simulink model "FOC_PMSM"  (Simulink 10.0)
settings: Solver=ode45  StartTime=0  StopTime=10  FixedStep=1/fs/4  MaxStep=1/fs/2  RelTol=1e-7  EnableMultiTasking=on
InitFcn:
  | Motor_parameters_Lsrpm7fw
values from neighbouring files (symbols this model uses):
  c2 = -L2/(L1^2-L2^2)    (= 10.9375)    [Motor_parameters_Lsrpm7fw.m]
  fs = 10e3    (= 10000)    [Motor_parameters_Lsrpm7fw.m]
  Iphmax = I_rated*sqrt(2)*3    [Motor_parameters_Lsrpm7fw.m]
  J = 1*1e-3    (= 0.001)    [Motor_parameters_Lsrpm7fw.m]
  Ki1 = 2    [Motor_parameters_Lsrpm7fw.m]
  Ki2 = 10000    [Motor_parameters_Lsrpm7fw.m]
  Ki_pll = 100    [Motor_parameters_Lsrpm7fw.m]
  Kp1 = 0.05    [Motor_parameters_Lsrpm7fw.m]
  Kp2 = 12    [Motor_parameters_Lsrpm7fw.m]
  Kp_pll = 10    [Motor_parameters_Lsrpm7fw.m]
  Ld = 10e-3    (= 0.01)    [Motor_parameters_Lsrpm7fw.m]
  Lndd_ini = Lndmpm    (= 0.412)    [Motor_parameters_Lsrpm7fw.m]
  Lndmpm = 0.412    [Motor_parameters_Lsrpm7fw.m]
  Lq = 12.8e-3    (= 0.0128)    [Motor_parameters_Lsrpm7fw.m]
  Npp = 8/2    (= 4)    [Motor_parameters_Lsrpm7fw.m]
  Omegae_ini = 0    [Motor_parameters_Lsrpm7fw.m]
  Rs = 0.78    [Motor_parameters_Lsrpm7fw.m]
  Tl_const = Trat/nrat^2    (= 1.24081632653e-05)    [Motor_parameters_Lsrpm7fw.m]
  Trat = 38    [Motor_parameters_Lsrpm7fw.m]
  Vm = 45    [Motor_parameters_Lsrpm7fw.m]
  Vph = Vs*sqrt(2)    [Motor_parameters_Lsrpm7fw.m]
  wo = 10    [Motor_parameters_Lsrpm7fw.m]
undefined symbols (not defined in the file or in its folder): DiscIntNeverNeededParam, sigbuilder_block
libraries: simulink x1
(part 2 of 2)

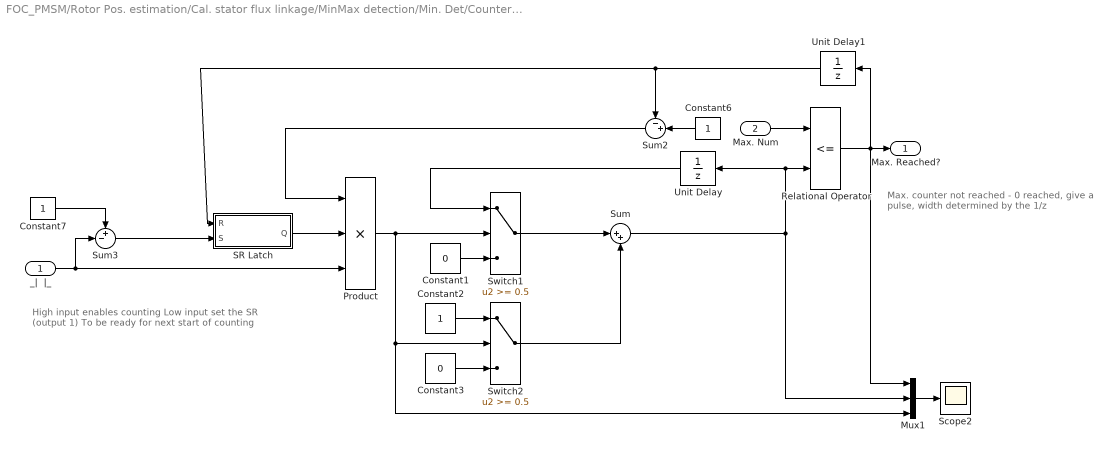
== system FOC_PMSM/Rotor Pos. estimation/Cal. stator flux linkage/MinMax detection/Min. Det/Counter.1/Conter with enable ==
  note: Max. counter not reached - 0
      | reached, give a pulse, width
      | determined by the 1/z
  note: High input enables counting
      | Low input set the SR (output 1)
      | To be ready for next start of
      | counting
  _|  |_ : Inport
  Max. Num : Inport  Port=2
  Constant1 : Constant  Value=0
  Constant2 : Constant
  Constant3 : Constant  Value=0
  Constant6 : Constant
  Constant7 : Constant
  Mux1 : Mux  Inputs=3
  Product : Product  Inputs=3  RndMeth=Zero
  Relational Operator : RelationalOperator  Operator=<=  RndMeth=Nearest
  SR Latch : Subsystem
  Scope2 : Scope
  Sum : Sum  Inputs=|++
  Sum2 : Sum  Inputs=-+|
  Sum3 : Sum  Inputs=+-|
  Switch1 : Switch  Threshold=0.5
  Switch2 : Switch  Threshold=0.5
  Unit Delay : UnitDelay  SampleTime=-1  HasFrameUpgradeWarning=on
  Unit Delay1 : UnitDelay  SampleTime=-1  HasFrameUpgradeWarning=on
  Max. Reached? : Outport  VectorParamsAs1DForOutWhenUnconnected=off
  wires:
  Unit Delay1/1 -> SR Latch/1(R), Sum2/1
  Constant6/1 -> Sum2/2
  Constant7/1 -> Sum3/1
  Sum3/1 -> SR Latch/2(S)
  SR Latch/1(Q) -> Product/2
  _|  |_/1 -> Product/3, Sum3/2
  Product/1 -> Mux1/3, Switch2/2, Switch1/2
  Sum2/1 -> Product/1
  Mux1/1 -> Scope2/1
  Relational Operator/1 -> Max. Reached?/1, Unit Delay1/1, Mux1/1
  Max. Num/1 -> Relational Operator/1
  Unit Delay/1 -> Switch1/1
  Sum/1 -> Mux1/2, Relational Operator/2, Unit Delay/1
  Switch2/1 -> Sum/2
  Switch1/1 -> Sum/1
  Constant3/1 -> Switch2/3
  Constant2/1 -> Switch2/1
  Constant1/1 -> Switch1/3

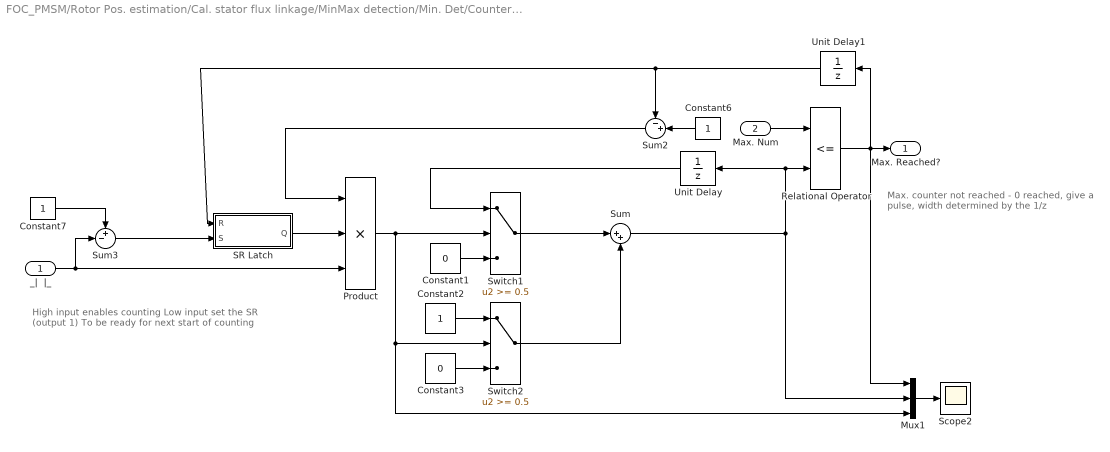
== system FOC_PMSM/Rotor Pos. estimation/Cal. stator flux linkage/MinMax detection/Min. Det/Counter.2/Conter with enable ==
  note: High input enables counting
      | Low input set the SR (output 1)
      | To be ready for next start of
      | counting
  note: Max. counter not reached - 0
      | reached, give a pulse, width
      | determined by the 1/z
  _|  |_ : Inport
  Max. Num : Inport  Port=2
  Constant1 : Constant  Value=0
  Constant2 : Constant
  Constant3 : Constant  Value=0
  Constant6 : Constant
  Constant7 : Constant
  Mux1 : Mux  Inputs=3
  Product : Product  Inputs=3  RndMeth=Zero
  Relational Operator : RelationalOperator  Operator=<=  RndMeth=Nearest
  SR Latch : Subsystem
  Scope2 : Scope
  Sum : Sum  Inputs=|++
  Sum2 : Sum  Inputs=-+|
  Sum3 : Sum  Inputs=+-|
  Switch1 : Switch  Threshold=0.5
  Switch2 : Switch  Threshold=0.5
  Unit Delay : UnitDelay  SampleTime=-1  HasFrameUpgradeWarning=on
  Unit Delay1 : UnitDelay  SampleTime=-1  HasFrameUpgradeWarning=on
  Max. Reached? : Outport  VectorParamsAs1DForOutWhenUnconnected=off
  wires:
  Constant1/1 -> Switch1/3
  Constant2/1 -> Switch2/1
  Constant3/1 -> Switch2/3
  Switch1/1 -> Sum/1
  Switch2/1 -> Sum/2
  Sum/1 -> Unit Delay/1, Relational Operator/2, Mux1/2
  Unit Delay/1 -> Switch1/1
  Max. Num/1 -> Relational Operator/1
  Relational Operator/1 -> Mux1/1, Unit Delay1/1, Max. Reached?/1
  Mux1/1 -> Scope2/1
  Sum2/1 -> Product/1
  Product/1 -> Switch1/2, Switch2/2, Mux1/3
  _|  |_/1 -> Sum3/2, Product/3
  SR Latch/1(Q) -> Product/2
  Sum3/1 -> SR Latch/2(S)
  Constant7/1 -> Sum3/1
  Constant6/1 -> Sum2/2
  Unit Delay1/1 -> Sum2/1, SR Latch/1(R)

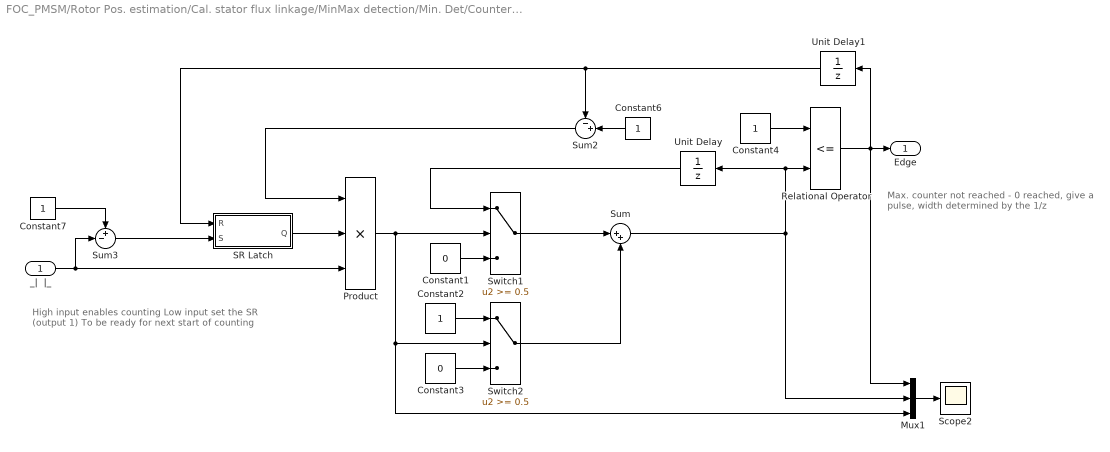
== system FOC_PMSM/Rotor Pos. estimation/Cal. stator flux linkage/MinMax detection/Min. Det/Counter.2/Rising edge gen. ==
  note: Max. counter not reached - 0
      | reached, give a pulse, width
      | determined by the 1/z
  note: High input enables counting
      | Low input set the SR (output 1)
      | To be ready for next start of
      | counting
  _|  |_ : Inport
  Constant1 : Constant  Value=0
  Constant{2,4,6..7} (4 alike) : Constant
  Constant3 : Constant  Value=0
  Mux1 : Mux  Inputs=3
  Product : Product  Inputs=3  RndMeth=Zero
  Relational Operator : RelationalOperator  Operator=<=  RndMeth=Nearest
  SR Latch : Subsystem
  Scope2 : Scope
  Sum : Sum  Inputs=|++
  Sum2 : Sum  Inputs=-+|
  Sum3 : Sum  Inputs=+-|
  Switch1 : Switch  Threshold=0.5
  Switch2 : Switch  Threshold=0.5
  Unit Delay : UnitDelay  SampleTime=-1  HasFrameUpgradeWarning=on
  Unit Delay1 : UnitDelay  SampleTime=-1  HasFrameUpgradeWarning=on
  Edge : Outport  VectorParamsAs1DForOutWhenUnconnected=off
  wires:
  Unit Delay1/1 -> SR Latch/1(R), Sum2/1
  Constant6/1 -> Sum2/2
  Constant7/1 -> Sum3/1
  Sum3/1 -> SR Latch/2(S)
  SR Latch/1(Q) -> Product/2
  _|  |_/1 -> Product/3, Sum3/2
  Product/1 -> Mux1/3, Switch2/2, Switch1/2
  Sum2/1 -> Product/1
  Mux1/1 -> Scope2/1
  Relational Operator/1 -> Edge/1, Unit Delay1/1, Mux1/1
  Constant4/1 -> Relational Operator/1
  Unit Delay/1 -> Switch1/1
  Sum/1 -> Mux1/2, Relational Operator/2, Unit Delay/1
  Switch2/1 -> Sum/2
  Switch1/1 -> Sum/1
  Constant3/1 -> Switch2/3
  Constant2/1 -> Switch2/1
  Constant1/1 -> Switch1/3

== system FOC_PMSM/Rotor Pos. estimation/Cal. stator flux linkage/MinMax detection/Min. Det/Counter.2/SR Latch ==
  R : Inport
  S : Inport  Port=2
  Constant2 : Constant
  Constant4 : Constant  Value=0
  Constant5 : Constant  Value=0
  Multiport Switch : MultiPortSwitch  Inputs=4
  Mux1 : Mux  Inputs=2
  Selcect : Fcn  Expr=(1-u(1))*(1-u(2))+2*(1-u(1))*u(2)+3*u(1)*(1-u(2))+4*u(1)*u(2)
  Unit Delay2 : UnitDelay  SampleTime=-1  HasFrameUpgradeWarning=on
  Q : Outport  VectorParamsAs1DForOutWhenUnconnected=off
  wires:
  Multiport Switch/1 -> Q/1, Unit Delay2/1
  Selcect/1 -> Multiport Switch/1
  Mux1/1 -> Selcect/1
  Unit Delay2/1 -> Multiport Switch/2
  Constant2/1 -> Multiport Switch/3
  Constant4/1 -> Multiport Switch/4
  Constant5/1 -> Multiport Switch/5
  R/1 -> Mux1/1
  S/1 -> Mux1/2

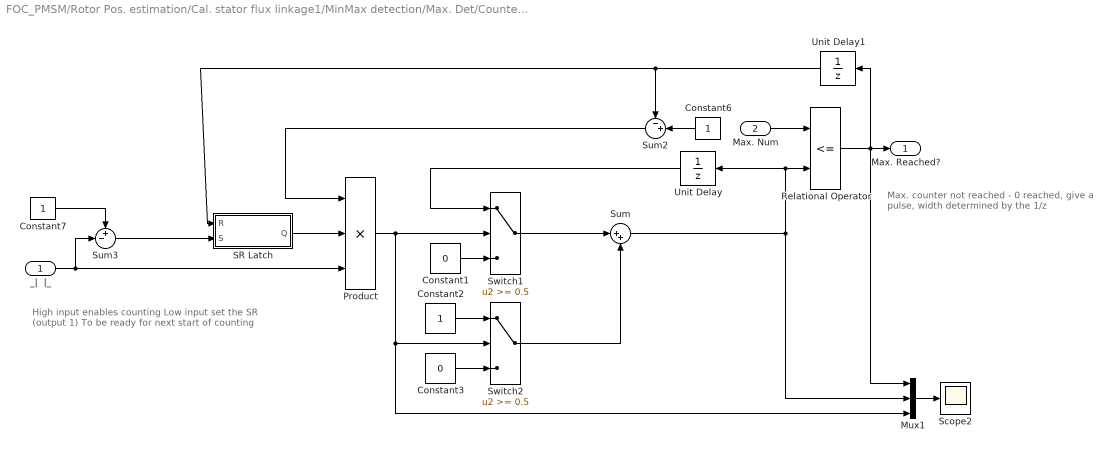
== system FOC_PMSM/Rotor Pos. estimation/Cal. stator flux linkage1/MinMax detection/Max. Det/Counter.1/Conter with enable ==
  note: High input enables counting
      | Low input set the SR (output 1)
      | To be ready for next start of
      | counting
  note: Max. counter not reached - 0
      | reached, give a pulse, width
      | determined by the 1/z
  _|  |_ : Inport
  Max. Num : Inport  Port=2
  Constant1 : Constant  Value=0
  Constant2 : Constant
  Constant3 : Constant  Value=0
  Constant6 : Constant
  Constant7 : Constant
  Mux1 : Mux  Inputs=3
  Product : Product  Inputs=3  RndMeth=Zero
  Relational Operator : RelationalOperator  Operator=<=  RndMeth=Nearest
  SR Latch : Subsystem
  Scope2 : Scope
  Sum : Sum  Inputs=|++
  Sum2 : Sum  Inputs=-+|
  Sum3 : Sum  Inputs=+-|
  Switch1 : Switch  Threshold=0.5
  Switch2 : Switch  Threshold=0.5
  Unit Delay : UnitDelay  SampleTime=-1  HasFrameUpgradeWarning=on
  Unit Delay1 : UnitDelay  SampleTime=-1  HasFrameUpgradeWarning=on
  Max. Reached? : Outport  VectorParamsAs1DForOutWhenUnconnected=off
  wires:
  Constant1/1 -> Switch1/3
  Constant2/1 -> Switch2/1
  Constant3/1 -> Switch2/3
  Switch1/1 -> Sum/1
  Switch2/1 -> Sum/2
  Sum/1 -> Unit Delay/1, Relational Operator/2, Mux1/2
  Unit Delay/1 -> Switch1/1
  Max. Num/1 -> Relational Operator/1
  Relational Operator/1 -> Mux1/1, Unit Delay1/1, Max. Reached?/1
  Mux1/1 -> Scope2/1
  Sum2/1 -> Product/1
  Product/1 -> Switch1/2, Switch2/2, Mux1/3
  _|  |_/1 -> Sum3/2, Product/3
  SR Latch/1(Q) -> Product/2
  Sum3/1 -> SR Latch/2(S)
  Constant7/1 -> Sum3/1
  Constant6/1 -> Sum2/2
  Unit Delay1/1 -> Sum2/1, SR Latch/1(R)

== system FOC_PMSM/Rotor Pos. estimation/Cal. stator flux linkage1/MinMax detection/Max. Det/Counter.2/Conter with enable ==
  note: Max. counter not reached - 0
      | reached, give a pulse, width
      | determined by the 1/z
  note: High input enables counting
      | Low input set the SR (output 1)
      | To be ready for next start of
      | counting
  _|  |_ : Inport
  Max. Num : Inport  Port=2
  Constant1 : Constant  Value=0
  Constant2 : Constant
  Constant3 : Constant  Value=0
  Constant6 : Constant
  Constant7 : Constant
  Mux1 : Mux  Inputs=3
  Product : Product  Inputs=3  RndMeth=Zero
  Relational Operator : RelationalOperator  Operator=<=  RndMeth=Nearest
  SR Latch : Subsystem
  Scope2 : Scope
  Sum : Sum  Inputs=|++
  Sum2 : Sum  Inputs=-+|
  Sum3 : Sum  Inputs=+-|
  Switch1 : Switch  Threshold=0.5
  Switch2 : Switch  Threshold=0.5
  Unit Delay : UnitDelay  SampleTime=-1  HasFrameUpgradeWarning=on
  Unit Delay1 : UnitDelay  SampleTime=-1  HasFrameUpgradeWarning=on
  Max. Reached? : Outport  VectorParamsAs1DForOutWhenUnconnected=off
  wires:
  Unit Delay1/1 -> SR Latch/1(R), Sum2/1
  Constant6/1 -> Sum2/2
  Constant7/1 -> Sum3/1
  Sum3/1 -> SR Latch/2(S)
  SR Latch/1(Q) -> Product/2
  _|  |_/1 -> Product/3, Sum3/2
  Product/1 -> Mux1/3, Switch2/2, Switch1/2
  Sum2/1 -> Product/1
  Mux1/1 -> Scope2/1
  Relational Operator/1 -> Max. Reached?/1, Unit Delay1/1, Mux1/1
  Max. Num/1 -> Relational Operator/1
  Unit Delay/1 -> Switch1/1
  Sum/1 -> Mux1/2, Relational Operator/2, Unit Delay/1
  Switch2/1 -> Sum/2
  Switch1/1 -> Sum/1
  Constant3/1 -> Switch2/3
  Constant2/1 -> Switch2/1
  Constant1/1 -> Switch1/3

== system FOC_PMSM/Rotor Pos. estimation/Cal. stator flux linkage1/MinMax detection/Max. Det/Counter.2/Rising edge gen. ==
  note: High input enables counting
      | Low input set the SR (output 1)
      | To be ready for next start of
      | counting
  note: Max. counter not reached - 0
      | reached, give a pulse, width
      | determined by the 1/z
  _|  |_ : Inport
  Constant1 : Constant  Value=0
  Constant{2,4,6..7} (4 alike) : Constant
  Constant3 : Constant  Value=0
  Mux1 : Mux  Inputs=3
  Product : Product  Inputs=3  RndMeth=Zero
  Relational Operator : RelationalOperator  Operator=<=  RndMeth=Nearest
  SR Latch : Subsystem
  Scope2 : Scope
  Sum : Sum  Inputs=|++
  Sum2 : Sum  Inputs=-+|
  Sum3 : Sum  Inputs=+-|
  Switch1 : Switch  Threshold=0.5
  Switch2 : Switch  Threshold=0.5
  Unit Delay : UnitDelay  SampleTime=-1  HasFrameUpgradeWarning=on
  Unit Delay1 : UnitDelay  SampleTime=-1  HasFrameUpgradeWarning=on
  Edge : Outport  VectorParamsAs1DForOutWhenUnconnected=off
  wires:
  Constant1/1 -> Switch1/3
  Constant2/1 -> Switch2/1
  Constant3/1 -> Switch2/3
  Switch1/1 -> Sum/1
  Switch2/1 -> Sum/2
  Sum/1 -> Unit Delay/1, Relational Operator/2, Mux1/2
  Unit Delay/1 -> Switch1/1
  Constant4/1 -> Relational Operator/1
  Relational Operator/1 -> Mux1/1, Unit Delay1/1, Edge/1
  Mux1/1 -> Scope2/1
  Sum2/1 -> Product/1
  Product/1 -> Switch1/2, Switch2/2, Mux1/3
  _|  |_/1 -> Sum3/2, Product/3
  SR Latch/1(Q) -> Product/2
  Sum3/1 -> SR Latch/2(S)
  Constant7/1 -> Sum3/1
  Constant6/1 -> Sum2/2
  Unit Delay1/1 -> Sum2/1, SR Latch/1(R)

== system FOC_PMSM/Rotor Pos. estimation/Cal. stator flux linkage1/MinMax detection/Max. Det/Counter.2/SR Latch ==
  R : Inport
  S : Inport  Port=2
  Constant2 : Constant
  Constant4 : Constant  Value=0
  Constant5 : Constant  Value=0
  Multiport Switch : MultiPortSwitch  Inputs=4
  Mux1 : Mux  Inputs=2
  Selcect : Fcn  Expr=(1-u(1))*(1-u(2))+2*(1-u(1))*u(2)+3*u(1)*(1-u(2))+4*u(1)*u(2)
  Unit Delay2 : UnitDelay  SampleTime=-1  HasFrameUpgradeWarning=on
  Q : Outport  VectorParamsAs1DForOutWhenUnconnected=off
  wires:
  S/1 -> Mux1/2
  R/1 -> Mux1/1
  Constant5/1 -> Multiport Switch/5
  Constant4/1 -> Multiport Switch/4
  Constant2/1 -> Multiport Switch/3
  Unit Delay2/1 -> Multiport Switch/2
  Mux1/1 -> Selcect/1
  Selcect/1 -> Multiport Switch/1
  Multiport Switch/1 -> Unit Delay2/1, Q/1

== system FOC_PMSM/Rotor Pos. estimation/Cal. stator flux linkage1/MinMax detection/Min. Det/Counter.1/Conter with enable ==
  note: Max. counter not reached - 0
      | reached, give a pulse, width
      | determined by the 1/z
  note: High input enables counting
      | Low input set the SR (output 1)
      | To be ready for next start of
      | counting
  _|  |_ : Inport
  Max. Num : Inport  Port=2
  Constant1 : Constant  Value=0
  Constant2 : Constant
  Constant3 : Constant  Value=0
  Constant6 : Constant
  Constant7 : Constant
  Mux1 : Mux  Inputs=3
  Product : Product  Inputs=3  RndMeth=Zero
  Relational Operator : RelationalOperator  Operator=<=  RndMeth=Nearest
  SR Latch : Subsystem
  Scope2 : Scope
  Sum : Sum  Inputs=|++
  Sum2 : Sum  Inputs=-+|
  Sum3 : Sum  Inputs=+-|
  Switch1 : Switch  Threshold=0.5
  Switch2 : Switch  Threshold=0.5
  Unit Delay : UnitDelay  SampleTime=-1  HasFrameUpgradeWarning=on
  Unit Delay1 : UnitDelay  SampleTime=-1  HasFrameUpgradeWarning=on
  Max. Reached? : Outport  VectorParamsAs1DForOutWhenUnconnected=off
  wires:
  Unit Delay1/1 -> SR Latch/1(R), Sum2/1
  Constant6/1 -> Sum2/2
  Constant7/1 -> Sum3/1
  Sum3/1 -> SR Latch/2(S)
  SR Latch/1(Q) -> Product/2
  _|  |_/1 -> Product/3, Sum3/2
  Product/1 -> Mux1/3, Switch2/2, Switch1/2
  Sum2/1 -> Product/1
  Mux1/1 -> Scope2/1
  Relational Operator/1 -> Max. Reached?/1, Unit Delay1/1, Mux1/1
  Max. Num/1 -> Relational Operator/1
  Unit Delay/1 -> Switch1/1
  Sum/1 -> Mux1/2, Relational Operator/2, Unit Delay/1
  Switch2/1 -> Sum/2
  Switch1/1 -> Sum/1
  Constant3/1 -> Switch2/3
  Constant2/1 -> Switch2/1
  Constant1/1 -> Switch1/3

== system FOC_PMSM/Rotor Pos. estimation/Cal. stator flux linkage1/MinMax detection/Min. Det/Counter.2/Conter with enable ==
  note: High input enables counting
      | Low input set the SR (output 1)
      | To be ready for next start of
      | counting
  note: Max. counter not reached - 0
      | reached, give a pulse, width
      | determined by the 1/z
  _|  |_ : Inport
  Max. Num : Inport  Port=2
  Constant1 : Constant  Value=0
  Constant2 : Constant
  Constant3 : Constant  Value=0
  Constant6 : Constant
  Constant7 : Constant
  Mux1 : Mux  Inputs=3
  Product : Product  Inputs=3  RndMeth=Zero
  Relational Operator : RelationalOperator  Operator=<=  RndMeth=Nearest
  SR Latch : Subsystem
  Scope2 : Scope
  Sum : Sum  Inputs=|++
  Sum2 : Sum  Inputs=-+|
  Sum3 : Sum  Inputs=+-|
  Switch1 : Switch  Threshold=0.5
  Switch2 : Switch  Threshold=0.5
  Unit Delay : UnitDelay  SampleTime=-1  HasFrameUpgradeWarning=on
  Unit Delay1 : UnitDelay  SampleTime=-1  HasFrameUpgradeWarning=on
  Max. Reached? : Outport  VectorParamsAs1DForOutWhenUnconnected=off
  wires:
  Constant1/1 -> Switch1/3
  Constant2/1 -> Switch2/1
  Constant3/1 -> Switch2/3
  Switch1/1 -> Sum/1
  Switch2/1 -> Sum/2
  Sum/1 -> Unit Delay/1, Relational Operator/2, Mux1/2
  Unit Delay/1 -> Switch1/1
  Max. Num/1 -> Relational Operator/1
  Relational Operator/1 -> Mux1/1, Unit Delay1/1, Max. Reached?/1
  Mux1/1 -> Scope2/1
  Sum2/1 -> Product/1
  Product/1 -> Switch1/2, Switch2/2, Mux1/3
  _|  |_/1 -> Sum3/2, Product/3
  SR Latch/1(Q) -> Product/2
  Sum3/1 -> SR Latch/2(S)
  Constant7/1 -> Sum3/1
  Constant6/1 -> Sum2/2
  Unit Delay1/1 -> Sum2/1, SR Latch/1(R)

== system FOC_PMSM/Rotor Pos. estimation/Cal. stator flux linkage1/MinMax detection/Min. Det/Counter.2/Rising edge gen. ==
  note: Max. counter not reached - 0
      | reached, give a pulse, width
      | determined by the 1/z
  note: High input enables counting
      | Low input set the SR (output 1)
      | To be ready for next start of
      | counting
  _|  |_ : Inport
  Constant1 : Constant  Value=0
  Constant{2,4,6..7} (4 alike) : Constant
  Constant3 : Constant  Value=0
  Mux1 : Mux  Inputs=3
  Product : Product  Inputs=3  RndMeth=Zero
  Relational Operator : RelationalOperator  Operator=<=  RndMeth=Nearest
  SR Latch : Subsystem
  Scope2 : Scope
  Sum : Sum  Inputs=|++
  Sum2 : Sum  Inputs=-+|
  Sum3 : Sum  Inputs=+-|
  Switch1 : Switch  Threshold=0.5
  Switch2 : Switch  Threshold=0.5
  Unit Delay : UnitDelay  SampleTime=-1  HasFrameUpgradeWarning=on
  Unit Delay1 : UnitDelay  SampleTime=-1  HasFrameUpgradeWarning=on
  Edge : Outport  VectorParamsAs1DForOutWhenUnconnected=off
  wires:
  Unit Delay1/1 -> SR Latch/1(R), Sum2/1
  Constant6/1 -> Sum2/2
  Constant7/1 -> Sum3/1
  Sum3/1 -> SR Latch/2(S)
  SR Latch/1(Q) -> Product/2
  _|  |_/1 -> Product/3, Sum3/2
  Product/1 -> Mux1/3, Switch2/2, Switch1/2
  Sum2/1 -> Product/1
  Mux1/1 -> Scope2/1
  Relational Operator/1 -> Edge/1, Unit Delay1/1, Mux1/1
  Constant4/1 -> Relational Operator/1
  Unit Delay/1 -> Switch1/1
  Sum/1 -> Mux1/2, Relational Operator/2, Unit Delay/1
  Switch2/1 -> Sum/2
  Switch1/1 -> Sum/1
  Constant3/1 -> Switch2/3
  Constant2/1 -> Switch2/1
  Constant1/1 -> Switch1/3

== system FOC_PMSM/Rotor Pos. estimation/Cal. stator flux linkage1/MinMax detection/Min. Det/Counter.2/SR Latch ==
  R : Inport
  S : Inport  Port=2
  Constant2 : Constant
  Constant4 : Constant  Value=0
  Constant5 : Constant  Value=0
  Multiport Switch : MultiPortSwitch  Inputs=4
  Mux1 : Mux  Inputs=2
  Selcect : Fcn  Expr=(1-u(1))*(1-u(2))+2*(1-u(1))*u(2)+3*u(1)*(1-u(2))+4*u(1)*u(2)
  Unit Delay2 : UnitDelay  SampleTime=-1  HasFrameUpgradeWarning=on
  Q : Outport  VectorParamsAs1DForOutWhenUnconnected=off
  wires:
  Multiport Switch/1 -> Q/1, Unit Delay2/1
  Selcect/1 -> Multiport Switch/1
  Mux1/1 -> Selcect/1
  Unit Delay2/1 -> Multiport Switch/2
  Constant2/1 -> Multiport Switch/3
  Constant4/1 -> Multiport Switch/4
  Constant5/1 -> Multiport Switch/5
  R/1 -> Mux1/1
  S/1 -> Mux1/2

== system FOC_PMSM/Rotor Pos. estimation/Cal. stator flux linkage/MinMax detection/Max. Det/Counter.1/Conter with enable/SR Latch ==
  R : Inport
  S : Inport  Port=2
  Constant2 : Constant
  Constant4 : Constant  Value=0
  Constant5 : Constant  Value=0
  Multiport Switch : MultiPortSwitch  Inputs=4
  Mux1 : Mux  Inputs=2
  Selcect : Fcn  Expr=(1-u(1))*(1-u(2))+2*(1-u(1))*u(2)+3*u(1)*(1-u(2))+4*u(1)*u(2)
  Unit Delay2 : UnitDelay  SampleTime=-1  HasFrameUpgradeWarning=on
  Q : Outport  VectorParamsAs1DForOutWhenUnconnected=off
  wires:
  Multiport Switch/1 -> Q/1, Unit Delay2/1
  Selcect/1 -> Multiport Switch/1
  Mux1/1 -> Selcect/1
  Unit Delay2/1 -> Multiport Switch/2
  Constant2/1 -> Multiport Switch/3
  Constant4/1 -> Multiport Switch/4
  Constant5/1 -> Multiport Switch/5
  R/1 -> Mux1/1
  S/1 -> Mux1/2

== system FOC_PMSM/Rotor Pos. estimation/Cal. stator flux linkage/MinMax detection/Max. Det/Counter.2/Conter with enable/SR Latch ==
  R : Inport
  S : Inport  Port=2
  Constant2 : Constant
  Constant4 : Constant  Value=0
  Constant5 : Constant  Value=0
  Multiport Switch : MultiPortSwitch  Inputs=4
  Mux1 : Mux  Inputs=2
  Selcect : Fcn  Expr=(1-u(1))*(1-u(2))+2*(1-u(1))*u(2)+3*u(1)*(1-u(2))+4*u(1)*u(2)
  Unit Delay2 : UnitDelay  SampleTime=-1  HasFrameUpgradeWarning=on
  Q : Outport  VectorParamsAs1DForOutWhenUnconnected=off
  wires:
  S/1 -> Mux1/2
  R/1 -> Mux1/1
  Constant5/1 -> Multiport Switch/5
  Constant4/1 -> Multiport Switch/4
  Constant2/1 -> Multiport Switch/3
  Unit Delay2/1 -> Multiport Switch/2
  Mux1/1 -> Selcect/1
  Selcect/1 -> Multiport Switch/1
  Multiport Switch/1 -> Unit Delay2/1, Q/1

== system FOC_PMSM/Rotor Pos. estimation/Cal. stator flux linkage/MinMax detection/Max. Det/Counter.2/Rising edge gen./SR Latch ==
  R : Inport
  S : Inport  Port=2
  Constant2 : Constant
  Constant4 : Constant  Value=0
  Constant5 : Constant  Value=0
  Multiport Switch : MultiPortSwitch  Inputs=4
  Mux1 : Mux  Inputs=2
  Selcect : Fcn  Expr=(1-u(1))*(1-u(2))+2*(1-u(1))*u(2)+3*u(1)*(1-u(2))+4*u(1)*u(2)
  Unit Delay2 : UnitDelay  SampleTime=-1  HasFrameUpgradeWarning=on
  Q : Outport  VectorParamsAs1DForOutWhenUnconnected=off
  wires:
  Multiport Switch/1 -> Q/1, Unit Delay2/1
  Selcect/1 -> Multiport Switch/1
  Mux1/1 -> Selcect/1
  Unit Delay2/1 -> Multiport Switch/2
  Constant2/1 -> Multiport Switch/3
  Constant4/1 -> Multiport Switch/4
  Constant5/1 -> Multiport Switch/5
  R/1 -> Mux1/1
  S/1 -> Mux1/2

== system FOC_PMSM/Rotor Pos. estimation/Cal. stator flux linkage/MinMax detection/Min. Det/Counter.1/Conter with enable/SR Latch ==
  R : Inport
  S : Inport  Port=2
  Constant2 : Constant
  Constant4 : Constant  Value=0
  Constant5 : Constant  Value=0
  Multiport Switch : MultiPortSwitch  Inputs=4
  Mux1 : Mux  Inputs=2
  Selcect : Fcn  Expr=(1-u(1))*(1-u(2))+2*(1-u(1))*u(2)+3*u(1)*(1-u(2))+4*u(1)*u(2)
  Unit Delay2 : UnitDelay  SampleTime=-1  HasFrameUpgradeWarning=on
  Q : Outport  VectorParamsAs1DForOutWhenUnconnected=off
  wires:
  S/1 -> Mux1/2
  R/1 -> Mux1/1
  Constant5/1 -> Multiport Switch/5
  Constant4/1 -> Multiport Switch/4
  Constant2/1 -> Multiport Switch/3
  Unit Delay2/1 -> Multiport Switch/2
  Mux1/1 -> Selcect/1
  Selcect/1 -> Multiport Switch/1
  Multiport Switch/1 -> Unit Delay2/1, Q/1

== system FOC_PMSM/Rotor Pos. estimation/Cal. stator flux linkage/MinMax detection/Min. Det/Counter.2/Conter with enable/SR Latch ==
  R : Inport
  S : Inport  Port=2
  Constant2 : Constant
  Constant4 : Constant  Value=0
  Constant5 : Constant  Value=0
  Multiport Switch : MultiPortSwitch  Inputs=4
  Mux1 : Mux  Inputs=2
  Selcect : Fcn  Expr=(1-u(1))*(1-u(2))+2*(1-u(1))*u(2)+3*u(1)*(1-u(2))+4*u(1)*u(2)
  Unit Delay2 : UnitDelay  SampleTime=-1  HasFrameUpgradeWarning=on
  Q : Outport  VectorParamsAs1DForOutWhenUnconnected=off
  wires:
  Multiport Switch/1 -> Q/1, Unit Delay2/1
  Selcect/1 -> Multiport Switch/1
  Mux1/1 -> Selcect/1
  Unit Delay2/1 -> Multiport Switch/2
  Constant2/1 -> Multiport Switch/3
  Constant4/1 -> Multiport Switch/4
  Constant5/1 -> Multiport Switch/5
  R/1 -> Mux1/1
  S/1 -> Mux1/2

== system FOC_PMSM/Rotor Pos. estimation/Cal. stator flux linkage/MinMax detection/Min. Det/Counter.2/Rising edge gen./SR Latch ==
  R : Inport
  S : Inport  Port=2
  Constant2 : Constant
  Constant4 : Constant  Value=0
  Constant5 : Constant  Value=0
  Multiport Switch : MultiPortSwitch  Inputs=4
  Mux1 : Mux  Inputs=2
  Selcect : Fcn  Expr=(1-u(1))*(1-u(2))+2*(1-u(1))*u(2)+3*u(1)*(1-u(2))+4*u(1)*u(2)
  Unit Delay2 : UnitDelay  SampleTime=-1  HasFrameUpgradeWarning=on
  Q : Outport  VectorParamsAs1DForOutWhenUnconnected=off
  wires:
  S/1 -> Mux1/2
  R/1 -> Mux1/1
  Constant5/1 -> Multiport Switch/5
  Constant4/1 -> Multiport Switch/4
  Constant2/1 -> Multiport Switch/3
  Unit Delay2/1 -> Multiport Switch/2
  Mux1/1 -> Selcect/1
  Selcect/1 -> Multiport Switch/1
  Multiport Switch/1 -> Unit Delay2/1, Q/1

== system FOC_PMSM/Rotor Pos. estimation/Cal. stator flux linkage1/MinMax detection/Max. Det/Counter.1/Conter with enable/SR Latch ==
  R : Inport
  S : Inport  Port=2
  Constant2 : Constant
  Constant4 : Constant  Value=0
  Constant5 : Constant  Value=0
  Multiport Switch : MultiPortSwitch  Inputs=4
  Mux1 : Mux  Inputs=2
  Selcect : Fcn  Expr=(1-u(1))*(1-u(2))+2*(1-u(1))*u(2)+3*u(1)*(1-u(2))+4*u(1)*u(2)
  Unit Delay2 : UnitDelay  SampleTime=-1  HasFrameUpgradeWarning=on
  Q : Outport  VectorParamsAs1DForOutWhenUnconnected=off
  wires:
  Multiport Switch/1 -> Q/1, Unit Delay2/1
  Selcect/1 -> Multiport Switch/1
  Mux1/1 -> Selcect/1
  Unit Delay2/1 -> Multiport Switch/2
  Constant2/1 -> Multiport Switch/3
  Constant4/1 -> Multiport Switch/4
  Constant5/1 -> Multiport Switch/5
  R/1 -> Mux1/1
  S/1 -> Mux1/2

== system FOC_PMSM/Rotor Pos. estimation/Cal. stator flux linkage1/MinMax detection/Max. Det/Counter.2/Conter with enable/SR Latch ==
  R : Inport
  S : Inport  Port=2
  Constant2 : Constant
  Constant4 : Constant  Value=0
  Constant5 : Constant  Value=0
  Multiport Switch : MultiPortSwitch  Inputs=4
  Mux1 : Mux  Inputs=2
  Selcect : Fcn  Expr=(1-u(1))*(1-u(2))+2*(1-u(1))*u(2)+3*u(1)*(1-u(2))+4*u(1)*u(2)
  Unit Delay2 : UnitDelay  SampleTime=-1  HasFrameUpgradeWarning=on
  Q : Outport  VectorParamsAs1DForOutWhenUnconnected=off
  wires:
  S/1 -> Mux1/2
  R/1 -> Mux1/1
  Constant5/1 -> Multiport Switch/5
  Constant4/1 -> Multiport Switch/4
  Constant2/1 -> Multiport Switch/3
  Unit Delay2/1 -> Multiport Switch/2
  Mux1/1 -> Selcect/1
  Selcect/1 -> Multiport Switch/1
  Multiport Switch/1 -> Unit Delay2/1, Q/1

== system FOC_PMSM/Rotor Pos. estimation/Cal. stator flux linkage1/MinMax detection/Max. Det/Counter.2/Rising edge gen./SR Latch ==
  R : Inport
  S : Inport  Port=2
  Constant2 : Constant
  Constant4 : Constant  Value=0
  Constant5 : Constant  Value=0
  Multiport Switch : MultiPortSwitch  Inputs=4
  Mux1 : Mux  Inputs=2
  Selcect : Fcn  Expr=(1-u(1))*(1-u(2))+2*(1-u(1))*u(2)+3*u(1)*(1-u(2))+4*u(1)*u(2)
  Unit Delay2 : UnitDelay  SampleTime=-1  HasFrameUpgradeWarning=on
  Q : Outport  VectorParamsAs1DForOutWhenUnconnected=off
  wires:
  Multiport Switch/1 -> Q/1, Unit Delay2/1
  Selcect/1 -> Multiport Switch/1
  Mux1/1 -> Selcect/1
  Unit Delay2/1 -> Multiport Switch/2
  Constant2/1 -> Multiport Switch/3
  Constant4/1 -> Multiport Switch/4
  Constant5/1 -> Multiport Switch/5
  R/1 -> Mux1/1
  S/1 -> Mux1/2

== system FOC_PMSM/Rotor Pos. estimation/Cal. stator flux linkage1/MinMax detection/Min. Det/Counter.1/Conter with enable/SR Latch ==
  R : Inport
  S : Inport  Port=2
  Constant2 : Constant
  Constant4 : Constant  Value=0
  Constant5 : Constant  Value=0
  Multiport Switch : MultiPortSwitch  Inputs=4
  Mux1 : Mux  Inputs=2
  Selcect : Fcn  Expr=(1-u(1))*(1-u(2))+2*(1-u(1))*u(2)+3*u(1)*(1-u(2))+4*u(1)*u(2)
  Unit Delay2 : UnitDelay  SampleTime=-1  HasFrameUpgradeWarning=on
  Q : Outport  VectorParamsAs1DForOutWhenUnconnected=off
  wires:
  S/1 -> Mux1/2
  R/1 -> Mux1/1
  Constant5/1 -> Multiport Switch/5
  Constant4/1 -> Multiport Switch/4
  Constant2/1 -> Multiport Switch/3
  Unit Delay2/1 -> Multiport Switch/2
  Mux1/1 -> Selcect/1
  Selcect/1 -> Multiport Switch/1
  Multiport Switch/1 -> Unit Delay2/1, Q/1

== system FOC_PMSM/Rotor Pos. estimation/Cal. stator flux linkage1/MinMax detection/Min. Det/Counter.2/Conter with enable/SR Latch ==
  R : Inport
  S : Inport  Port=2
  Constant2 : Constant
  Constant4 : Constant  Value=0
  Constant5 : Constant  Value=0
  Multiport Switch : MultiPortSwitch  Inputs=4
  Mux1 : Mux  Inputs=2
  Selcect : Fcn  Expr=(1-u(1))*(1-u(2))+2*(1-u(1))*u(2)+3*u(1)*(1-u(2))+4*u(1)*u(2)
  Unit Delay2 : UnitDelay  SampleTime=-1  HasFrameUpgradeWarning=on
  Q : Outport  VectorParamsAs1DForOutWhenUnconnected=off
  wires:
  Multiport Switch/1 -> Q/1, Unit Delay2/1
  Selcect/1 -> Multiport Switch/1
  Mux1/1 -> Selcect/1
  Unit Delay2/1 -> Multiport Switch/2
  Constant2/1 -> Multiport Switch/3
  Constant4/1 -> Multiport Switch/4
  Constant5/1 -> Multiport Switch/5
  R/1 -> Mux1/1
  S/1 -> Mux1/2

== system FOC_PMSM/Rotor Pos. estimation/Cal. stator flux linkage1/MinMax detection/Min. Det/Counter.2/Rising edge gen./SR Latch ==
  R : Inport
  S : Inport  Port=2
  Constant2 : Constant
  Constant4 : Constant  Value=0
  Constant5 : Constant  Value=0
  Multiport Switch : MultiPortSwitch  Inputs=4
  Mux1 : Mux  Inputs=2
  Selcect : Fcn  Expr=(1-u(1))*(1-u(2))+2*(1-u(1))*u(2)+3*u(1)*(1-u(2))+4*u(1)*u(2)
  Unit Delay2 : UnitDelay  SampleTime=-1  HasFrameUpgradeWarning=on
  Q : Outport  VectorParamsAs1DForOutWhenUnconnected=off
  wires:
  S/1 -> Mux1/2
  R/1 -> Mux1/1
  Constant5/1 -> Multiport Switch/5
  Constant4/1 -> Multiport Switch/4
  Constant2/1 -> Multiport Switch/3
  Unit Delay2/1 -> Multiport Switch/2
  Mux1/1 -> Selcect/1
  Selcect/1 -> Multiport Switch/1
  Multiport Switch/1 -> Unit Delay2/1, Q/1
